simulink model "VLC_OFDM"  (R2015b)
settings: Solver=FixedStepDiscrete  SolverMode=SingleTasking  StartTime=0.0  StopTime=1024  RelTol=1e-3
InitFcn:
  | wordLength = 13;
  | fracLength  = 6;
libraries: dspobslib x3, commdigbbndam3 x2, dspstat3 x1, dspxfrm3 x1, commseqgen2 x1, dspindex x1, commrandsrc2 x1
Description:
  | OFDM Receiver with 512-Point Streaming I/O FFT
  | This model shows how to use Simulink(R) HDL Coder(TM) to check, generate,
  | and verify HDL code for a 512-point streaming I/O DIF FFT block.
settings Model: FPTRunName=Active  Creator=mdonovan  LastModifiedBy=DELL
settings DataIOCC: SaveFormat=Array  SignalLoggingSaveFormat=ModelDataLogs  SaveOutput=off  SaveTime=off
settings OptimizationCC: BlockReduction=off  ConditionallyExecuteInputs=off  DefaultParameterBehavior=Inlined  ExpressionDepthLimit=2147483647  InitFltsAndDblsToZero=on  EfficientMapNaN2IntZero=off
settings DebuggingCC: AlgebraicLoopMsg=error  UnderspecifiedInitializationDetection=Classic  MergeDetectMultiDrivingBlocksExec=none  SolverPrmCheckMsg=warning  MultiTaskDSMMsg=warning  MultiTaskCondExecSysMsg=none  SingleTaskRateTransMsg=error  IntegerOverflowMsg=none  FcnCallInpInsideContextMsg=UseLocalSettings  StateNameClashWarn=warning  IntegerSaturationMsg=none
settings HardwareCC: ProdBitPerPointer=32  ProdLargestAtomicFloat=None  ProdIntDivRoundTo=Undefined  ProdEndianess=Unspecified  ProdWordSize=32  ProdHWDeviceType=ASIC/FPGA->ASIC/FPGA  ProdEqTarget=off
settings GRTTargetCC: GeneratePreprocessorConditionals=Disable all  CombineOutputUpdateFcns=off  GRTInterface=on
settings ConfigComp: CovModelRefEnable=Off  CovSFcnEnable=off

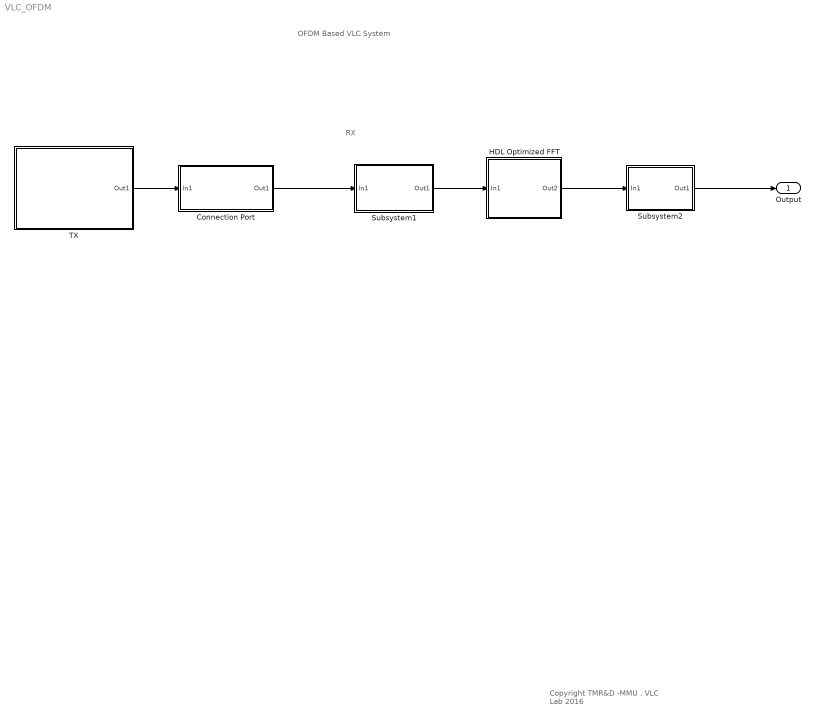
== system VLC_OFDM ==
  note: OFDM Based VLC System
  note: RX
  note: Copyright TMR&D -MMU .
      | VLC Lab
      | 2016
  Connection Port : Subsystem  TreatAsAtomicUnit=on
  HDL Optimized FFT : Subsystem
  Subsystem1 : Subsystem
  Subsystem2 : Subsystem
  TX : Subsystem
  "Output " : Outport
  wires:
  Connection Port/1(Out1) -> Subsystem1/1(In1)
  Subsystem1/1(Out1) -> HDL Optimized FFT/1(In1)
  HDL Optimized FFT/1(Out2) -> Subsystem2/1(In1)
  Subsystem2/1(Out1) -> "Output "/1
  TX/1(Out1) -> Connection Port/1(In1)

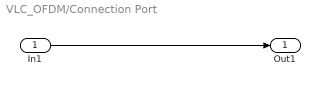
== system VLC_OFDM/Connection Port ==
  In1 : Inport
  Out1 : Outport
  wires:
  In1/1 -> Out1/1

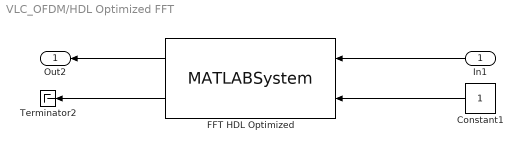
== system VLC_OFDM/HDL Optimized FFT ==
  In1 : Inport
  Constant1 : Constant  OutDataTypeStr=boolean  SampleTime=1
  FFT HDL Optimized : MATLABSystem  System=dsp.HDLFFT  BitReversedOutput=off  Normalize=off  FFTLengthSource=Property  FFTLength=512  RoundingMethod=Floor  OverflowAction=Saturate  ValidInputPort=on  ResetInputPort=off  StartOutputPort=off  EndOutputPort=off  SimulateUsing=Code generation
      mask Type: FFT HDL Optimized
      mask Display:
      | disp(['FFT' char(10) 'HDL Optimized' char(10) 'Latency = 1077']);
      | port_label('input',1,'dataIn');
      | port_label('input',2,'validIn');
      | port_label('output',1,'dataOut');
      | port_label('output',2,'validOut');
  Terminator2 : Terminator
  Out2 : Outport
  wires:
  In1/1 -> FFT HDL Optimized/1
  Constant1/1 -> FFT HDL Optimized/2
  FFT HDL Optimized/1 -> Out2/1
  FFT HDL Optimized/2 -> Terminator2/1

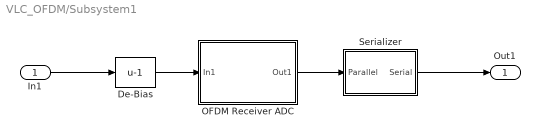
== system VLC_OFDM/Subsystem1 ==
  In1 : Inport
  De-Bias : Bias  Bias=-1
  OFDM Receiver ADC : Subsystem
  Serializer : Subsystem  mask(Serializer){}
      mask help: Serializer
  Out1 : Outport
  wires:
  Serializer/1(Serial) -> Out1/1
  OFDM Receiver ADC/1(Out1) -> Serializer/1(Parallel)
  De-Bias/1 -> OFDM Receiver ADC/1(In1)
  In1/1 -> De-Bias/1

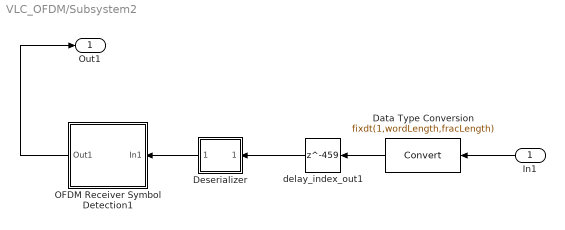
== system VLC_OFDM/Subsystem2 ==
  In1 : Inport
  Data Type Conversion : DataTypeConversion  OutDataTypeStr=fixdt(1,wordLength,fracLength)
  Deserializer : Subsystem  mask(DeSerializer){N=512}
      mask prompts: N "Output buffer size"
      mask help: DeSerializer
  OFDM Receiver Symbol Detection1 : Subsystem
  delay_index_out1 : Delay  DelayLength=459  InputProcessing=Inherited
  Out1 : Outport
  wires:
  OFDM Receiver Symbol Detection1/1(Out1) -> Out1/1
  delay_index_out1/1 -> Deserializer/1(Serial)
  Deserializer/1(Parallel) -> OFDM Receiver Symbol Detection1/1(In1)
  In1/1 -> Data Type Conversion/1
  Data Type Conversion/1 -> delay_index_out1/1

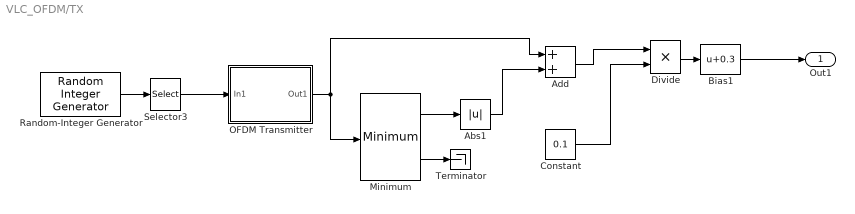
== system VLC_OFDM/TX ==
  Abs1 : Abs
  Add : Sum
  Bias1 : Bias  Bias=0.3
  Constant : Constant  Value=0.1  VectorParams1D=off  SampleTime=-1
  Divide : Product  RndMeth=Zero
  Minimum : dspstat3/Minimum  fcn=Value and Index  reset=None  InputProcessing=Columns as channels (frame based)  indexBase=One  operateOver=Each column  Dimension=1  operation=minimum  roiEnable=off  roiType=Rectangles  roiPortion=Entire ROI  roiOutput=Individual statistics for each ROI  roiFlag=off  roundingMode=Floor  overflowMode=off
  OFDM Transmitter : Subsystem
  Random-Integer Generator : commrandsrc2/Random Integer Generator  mul=64  seed=1234573  Ts=1  frameBased=on  sampPerFrame=512  orient=off  outDataType=uint8
  Selector3 : Selector  InputPortWidth=512  IndexOptions=Index vector (dialog)  Indices=[1:384]  OutputSizes=1
  Terminator : Terminator
  Out1 : Outport
  wires:
  Random-Integer Generator/1 -> Selector3/1
  OFDM Transmitter/1(Out1) -> Add/1, Minimum/1
  Constant/1 -> Divide/2
  Minimum/1 -> Abs1/1
  Abs1/1 -> Add/2
  Bias1/1 -> Out1/1
  Add/1 -> Divide/1
  Minimum/2 -> Terminator/1
  Divide/1 -> Bias1/1
  Selector3/1 -> OFDM Transmitter/1(In1)

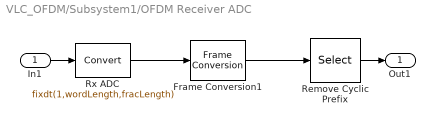
== system VLC_OFDM/Subsystem1/OFDM Receiver ADC ==
  In1 : Inport
  Frame Conversion1 : FrameConversion  InheritSamplingMode=off  OutFrame=Sample-based
  Remove Cyclic Prefix : Selector  NumberOfDimensions=2  InputPortWidth=80  IndexOptions=Index vector (dialog),Select all  Indices=[33:544],1  OutputSizes=1,1
  Rx ADC : DataTypeConversion  OutDataTypeStr=fixdt(1,wordLength,fracLength)
  Out1 : Outport
  wires:
  Rx ADC/1 -> Frame Conversion1/1
  Frame Conversion1/1 -> Remove Cyclic Prefix/1
  Remove Cyclic Prefix/1 -> Out1/1
  In1/1 -> Rx ADC/1

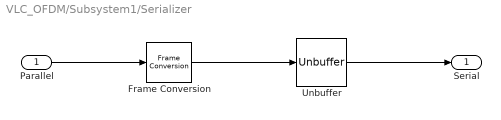
== system VLC_OFDM/Subsystem1/Serializer ==
  Parallel : Inport
  Frame Conversion : FrameConversion  InheritSamplingMode=off
  Unbuffer : Unbuffer  SampleBasedProcessing=Same as frame based
  Serial : Outport
  wires:
  Unbuffer/1 -> Serial/1
  Parallel/1 -> Frame Conversion/1
  Frame Conversion/1 -> Unbuffer/1

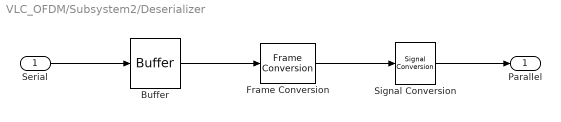
== system VLC_OFDM/Subsystem2/Deserializer ==
  Serial : Inport
  Buffer : Buffer  N=N  TreatMby1Signals=One channel
  Frame Conversion : FrameConversion  InheritSamplingMode=off  OutFrame=Sample-based
  Signal Conversion : SignalConversion  ConversionOutput=Contiguous copy
  Parallel : Outport
  wires:
  Signal Conversion/1 -> Parallel/1
  Frame Conversion/1 -> Signal Conversion/1
  Serial/1 -> Buffer/1
  Buffer/1 -> Frame Conversion/1

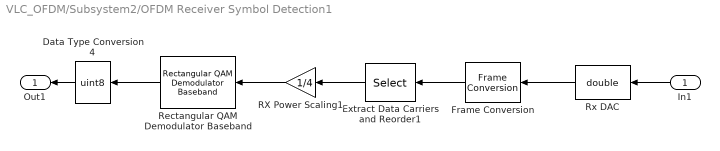
== system VLC_OFDM/Subsystem2/OFDM Receiver Symbol Detection1 ==
  In1 : Inport
  Data Type Conversion4 : DataTypeConversion  OutDataTypeStr=uint8
  Extract Data Carriers and Reorder1 : Selector  InputPortWidth=512  IndexOptions=Index vector (dialog)  Indices=[317:340 342:389 391:438 440:487 489:512 2:25 27:74 76:123 125:172 174:197]  OutputSizes=1
  Frame Conversion : FrameConversion  InheritSamplingMode=off
  RX Power Scaling1 : Gain  Gain=1/4
  Rectangular QAM Demodulator Baseband : commdigbbndam3/Rectangular QAM Demodulator Baseband  M=64  PowType=Min. distance between symbols  MinDist=2  AvgPow=1  PeakPow=1  Ph=0  Dec=Gray  Mapping=[0:15]  OutType=Integer  DecType=Hard decision  VarSource=Dialog  Variance=1  outDtype1=Inherit via internal rule  outDtype2=Inherit via internal rule  derotateFactorWordLen=16  denormFactorWordLen=16  prodOutWordLen=32  prodOutRoundingMode=Floor  prodOutOverflowMode=Wrap  sumWordLen=32
  Rx DAC : DataTypeConversion  OutDataTypeStr=double
  Out1 : Outport
  wires:
  In1/1 -> Rx DAC/1
  Data Type Conversion4/1 -> Out1/1
  Extract Data Carriers and Reorder1/1 -> RX Power Scaling1/1
  RX Power Scaling1/1 -> Rectangular QAM Demodulator Baseband/1
  Frame Conversion/1 -> Extract Data Carriers and Reorder1/1
  Rx DAC/1 -> Frame Conversion/1
  Rectangular QAM Demodulator Baseband/1 -> Data Type Conversion4/1

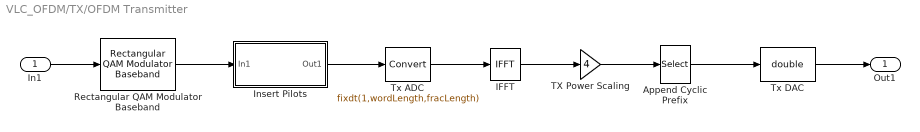
== system VLC_OFDM/TX/OFDM Transmitter ==
  In1 : Inport
  Append Cyclic Prefix : Selector  NumberOfDimensions=2  InputPortWidth=256  IndexOptions=Index vector (dialog),Select all  Indices=[481:512 1:512],1  OutputSizes=1,1
  IFFT : dspxfrm3/IFFT  FFTImplementation=Auto  CompMethod=Table lookup  TableOpt=HYBRID  TableOptActive=Speed  BitRevOrder=off  cs_in=on  Normalize=on  InheritFFTLength=on  FFTLength=64  WrapInput=on  mode=Complex  outSamplingMode=Frame based  roundingMode=Floor  overflowMode=off  firstCoeffMode=Specify word length  firstCoeffWordLength=16  firstCoeffFracLength=15  firstCoeffDataTypeStr=fixdt(1,16)  firstCoeffLastDataTypeStr=fixdt(1,16)  accumDataTypeStr=Inherit: Same as product output  accumLastDataTypeStr=Inherit: Same as product output  outputMin=[]  outputMax=[]
  Insert Pilots : Subsystem
  Rectangular QAM Modulator Baseband : commdigbbndam3/Rectangular QAM Modulator Baseband  M=64  InType=Integer  Enc=Gray  Mapping=[0:15]  PowType=Min. distance between symbols  MinDist=2  AvgPow=1  PeakPow=1  Ph=0  outDtype=double  outWordLen=16  outUDDataType=sfix(16)  outFracLenMode=Best precision  outFracLen=15
  TX Power Scaling : Gain  Gain=4
  Tx ADC : DataTypeConversion  OutDataTypeStr=fixdt(1,wordLength,fracLength)
  Tx DAC : DataTypeConversion  OutDataTypeStr=double
  Out1 : Outport
  wires:
  Rectangular QAM Modulator Baseband/1 -> Insert Pilots/1(In1)
  Insert Pilots/1(Out1) -> Tx ADC/1
  Tx ADC/1 -> IFFT/1
  TX Power Scaling/1 -> Append Cyclic Prefix/1
  IFFT/1 -> TX Power Scaling/1
  Append Cyclic Prefix/1 -> Tx DAC/1
  In1/1 -> Rectangular QAM Modulator Baseband/1
  Tx DAC/1 -> Out1/1

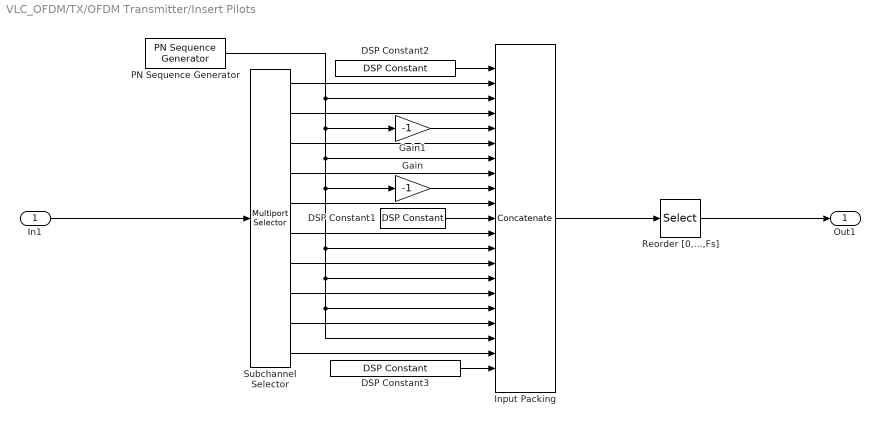
== system VLC_OFDM/TX/OFDM Transmitter/Insert Pilots ==
  In1 : Inport
  DSP Constant1 : dspobslib/DSP Constant  Value=complex(0,0)  SampleMode=Discrete  discreteOutput=Frame-based  continuousOutput=Sample-based  sampTime=1  framePeriod=inf  dataType=Inherit from 'Constant value'  isSigned=on  wordLen=16  udDataType=sfix(16)  fracBitsMode=Best precision  numFracBits=15  InterpretAs1D=-inf  Ts=-inf  FramebasedOutput=-inf
  DSP Constant2 : dspobslib/DSP Constant  Value=complex(zeros(60,1))  SampleMode=Discrete  discreteOutput=Frame-based  continuousOutput=Sample-based  sampTime=1  framePeriod=inf  dataType=Inherit from 'Constant value'  isSigned=on  wordLen=16  udDataType=sfix(16)  fracBitsMode=Best precision  numFracBits=15  InterpretAs1D=-inf  Ts=-inf  FramebasedOutput=-inf
  DSP Constant3 : dspobslib/DSP Constant  Value=complex(zeros(59,1))  SampleMode=Discrete  discreteOutput=Frame-based  continuousOutput=Sample-based  sampTime=1  framePeriod=inf  dataType=Inherit from 'Constant value'  isSigned=on  wordLen=16  udDataType=sfix(16)  fracBitsMode=Best precision  numFracBits=15  InterpretAs1D=-inf  Ts=-inf  FramebasedOutput=-inf
  Gain : Gain  Gain=-1
  Gain1 : Gain  Gain=-1
  Input Packing : Concatenate  NumInputs=21  Mode=Multidimensional array
  PN Sequence Generator : commseqgen2/PN Sequence Generator  poly=[1 0 0 0 0 0 0 0 0 0 0 0 0 1 1]  ini_sta=[1 0 0 1 0 1 0 1 0 0 0 0 0 0]  outBitMaskSource=Dialog parameter  shift=0  outVarSiz=off  maxOutSizeMode=Dialog parameter  maxOutSize=[10 1]  Ts=512  frameBased=on  sampPerFrame=1  reset=off  bitPackedOutputs=off  outDataType=double  numPackedBits=8  bitPackDataSigned=off  bitPackedOutDType=double
  Reorder [0,...,Fs] : Selector  NumberOfDimensions=2  InputPortWidth=256  IndexOptions=Index vector (dialog),Select all  Indices=[257:512 1:256],1  OutputSizes=1,1
  Subchannel Selector : dspindex/Multiport Selector  rowsOrCols=Rows  idxCellArray={[1:24],[25:72],[73:120],[121:168],[169:192],[193:216],[217:264],[265:312],[313:360],[361:384]}  idxErrMode=Generate Error
  Out1 : Outport
  wires:
  In1/1 -> Subchannel Selector/1
  PN Sequence Generator/1 -> Gain1/1, Gain/1, Input Packing/19, Input Packing/17, Input Packing/15, Input Packing/13, Input Packing/7, Input Packing/3
  Subchannel Selector/10 -> Input Packing/20
  Subchannel Selector/9 -> Input Packing/18
  Subchannel Selector/8 -> Input Packing/16
  Subchannel Selector/7 -> Input Packing/14
  Subchannel Selector/6 -> Input Packing/12
  Subchannel Selector/5 -> Input Packing/10
  Subchannel Selector/4 -> Input Packing/8
  Subchannel Selector/3 -> Input Packing/6
  Subchannel Selector/2 -> Input Packing/4
  Subchannel Selector/1 -> Input Packing/2
  DSP Constant1/1 -> Input Packing/11
  DSP Constant2/1 -> Input Packing/1
  DSP Constant3/1 -> Input Packing/21
  Gain/1 -> Input Packing/9
  Gain1/1 -> Input Packing/5
  Input Packing/1 -> Reorder [0,...,Fs]/1
  Reorder [0,...,Fs]/1 -> Out1/1
